simulink model "Pole_placement"  (R2023b)
settings: Solver=VariableStepAuto  StartTime=0.0  StopTime=30  RelTol=1e-3
values from neighbouring files (symbols this model uses):
  A = double(A)    [consistent.m]    (also in dyn_model.m)
  B = double(B)    [consistent.m]    (also in dyn_model.m; rot_pend.m = [a b)
  K = place(A,B,P)    [consistent.m]
  ss_gain = 1/dcgain(cl_lq)    [consistent.m]
  x1_bar = 0    [consistent.m]    (also in dyn_model.m)
  x3_bar = pi    (= 3.14159265359)    [consistent.m]    (also in dyn_model.m = 0)
libraries: simulink_extras x3
settings Model: Creator=Mark  LastModifiedBy=Mark

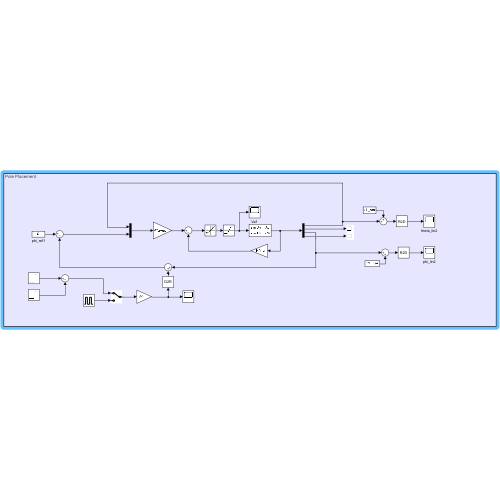
[thumbnail: Simulink's stored preview of the top-level diagram]
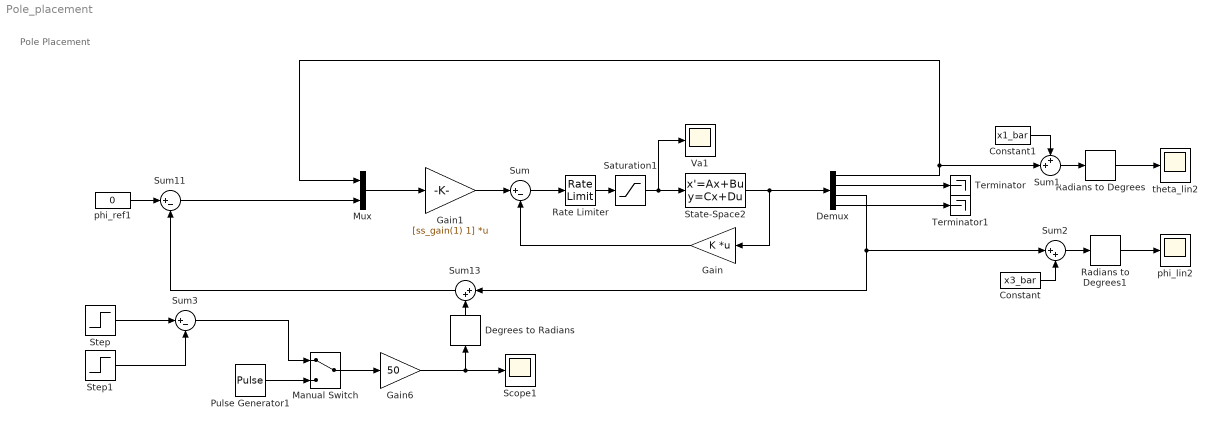
== system Pole_placement ==
  note: Pole Placement
  Constant : Constant  Value=x3_bar
  Constant1 : Constant  Value=x1_bar
  Degrees to Radians : simulink_extras/Transformations/Degrees to Radians
  Demux : Demux
  Gain : Gain  Gain=K  Multiplication=Matrix(K*u) (u vector)
  Gain1 : Gain  Gain=[ss_gain(1) 1]  Multiplication=Matrix(K*u) (u vector)
  Gain6 : Gain  Gain=50
  Manual Switch : ManualSwitch
  Mux : Mux  Inputs=2
  Pulse Generator1 : DiscretePulseGenerator  PulseType=Time based  Period=10000  PulseWidth=0.005  PhaseDelay=30
  Radians to Degrees : simulink_extras/Transformations/Radians to Degrees
  Radians to Degrees1 : simulink_extras/Transformations/Radians to Degrees
  Rate Limiter : RateLimiter  RisingSlewLimit=inf  FallingSlewLimit=-inf  SampleTimeMode=inherited
  Saturation1 : Saturate  UpperLimit=10  LowerLimit=-10
  Scope1 : Scope
  State-Space2 : StateSpace  A=A  B=B  C=[1 0 0 0; 0 1 0 0; 0 0 1 0; 0 0 0 1]  D=[0 0 0 0]'  InitialCondition=[0 0 0 0]
  Step : Step  Time=5  SampleTime=0
  Step1 : Step  Time=6  SampleTime=0
  Sum : Sum  Inputs=|+-
  Sum1 : Sum  Inputs=++|
  Sum11 : Sum  Inputs=|+-
  Sum13 : Sum  Inputs=|++
  Sum2 : Sum  Inputs=|++
  Sum3 : Sum  Inputs=|+-
  Terminator : Terminator
  Terminator1 : Terminator
  Va1 : Scope
  phi_lin2 : Scope
  phi_ref1 : Constant  Value=0
  theta_lin2 : Scope
  wires:
  phi_ref1/1 -> Sum11/1
  Sum11/1 -> Mux/2
  Demux/1 -> Sum1/2, Mux/1
  Pulse Generator1/1 -> Manual Switch/2
  Gain6/1 -> Scope1/1, Degrees to Radians/1
  Step/1 -> Sum3/1
  Radians to Degrees/1 -> theta_lin2/1
  Sum13/1 -> Sum11/2
  Manual Switch/1 -> Gain6/1
  State-Space2/1 -> Gain/1, Demux/1
  Gain/1 -> Sum/2
  Saturation1/1 -> Va1/1, State-Space2/1
  Demux/3 -> Sum2/1, Sum13/1
  Gain1/1 -> Sum/1
  Demux/2 -> Terminator/1
  Demux/4 -> Terminator1/1
  Mux/1 -> Gain1/1
  Sum/1 -> Rate Limiter/1
  Rate Limiter/1 -> Saturation1/1
  Radians to Degrees1/1 -> phi_lin2/1
  Degrees to Radians/1 -> Sum13/2
  Sum2/1 -> Radians to Degrees1/1
  Sum1/1 -> Radians to Degrees/1
  Constant/1 -> Sum2/2
  Constant1/1 -> Sum1/1
  Sum3/1 -> Manual Switch/1
  Step1/1 -> Sum3/2
